simulink library "per"  (Simulink 8.2)
settings: Solver=ode45  StartTime=0.0  StopTime=10.0  RelTol=1e-3
undefined symbols (not defined in the file or in its folder): C_TICK_TIME_S, ENUM_LANEQUALITY_HIGH, ENUM_LANEQUALITY_MEDIUM, ENUM_SENSORSTATE_NORMAL, FALSE, KAPP_VehicleWidth_m, KPER_C0CrossingThr_m, KPER_CalDefaultTLC_s, KPER_CalTLCMax_s, KPER_CalTLCMin_s, KPER_DefaultLaneWidth_m, KPER_LaneWidHoldOnTime_s, KPER_LaneWidRampFinErrThres_m, KPER_LaneWidRampFinTimeThres_s, KPER_LaneWidRampInFalRt_mps, KPER_LaneWidRampInRisRt_mps, KPER_LaneWidRampOutFalRt_mps, KPER_LaneWidRampOutRisRt_mps, KPER_TLCDefaultValue_s, KPER_UseCalTLC_flg, TRUE
libraries: hcu_lib x16, cam x1, rad x1, sdf x1
(part 1 of 2)
settings Model: Creator=xsellart  LastModifiedBy=14069

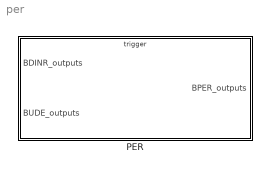
== system per ==
  PER : Subsystem

== system per/PER ==
  BDINR_outputs : Inport  OutDataTypeStr=Bus: BDINR_outputs
  BUDE_outputs : Inport  Port=2  OutDataTypeStr=Bus: BUDE_outputs
  trig_PER : TriggerPort  TriggerType=function-call
      settings: AttributesFormatString=State = %<StatesWhenEnabling>
  Bus Creator : BusCreator  Inputs=37  OutDataTypeStr=Bus: BPER_outputs
  Bus Selector1 : BusSelector  OutputSignals=VDINR_CamInternalError_flg,VDINR_LaneQualityL_enum,VDINR_LaneQualityR_enum,VDINR_LaneC0L_m,VDINR_LaneC0R_m,VDINR_LaneC1L_rad,VDINR_LaneC1R_rad,VDINR_LaneC2L_rat,VDINR_LaneC2R_rat,VDINR_LaneC3L_rat,VDINR_LaneC3R_rat,VDINR_TLCL_s,VDINR_TLCLValid_flg,VDINR_TLCR_s,VDINR_TLCRValid_flg,VDINR_VehSpd_mps,VDINR_YawRate_radps,VDINR_ViewRangeEndL_m,VDINR_ViewRangeEndR_m
  Bus Selector2 : BusSelector  OutputSignals=VUDE_NOFTRACKS_num,VUDE_TRACKSX_m,VUDE_TRACKSY_m,VUDE_TRACKSOBST_enum,VUDE_TRACKSVEL_mps,VUDE_TRACKSWIDTH_m,VUDE_TRACKSID_enum,VUDE_TRACKSATT_rad,VUDE_TRACKSEXSPROB_num,VUDE_TRACKSACCEL_mps2,VUDE_RadObjectValid_flg,VUDE_TRACKSRADDYNSTAT_enum,VUDE_CamObstacleValid_flg,VUDE_TRACKSMEDYNSTAT_enum
  per : Subsystem
  BPER_outputs : Outport  OutDataTypeStr=Bus: BPER_outputs
  wires:
  BDINR_outputs/1 -> Bus Selector1/1
  BUDE_outputs/1 -> Bus Selector2/1
  Bus Creator/1 -> BPER_outputs/1  "BPER_outputs"
  Bus Selector2/1 -> per/20(VUDE_NOfTracks_num)  "<VUDE_NOFTRACKS_num>"
  Bus Selector2/2 -> per/21(VUDE_TracksX_num)  "<VUDE_TRACKSX_m>"
  Bus Selector2/6 -> per/25(VUDE_TracksWidth_m)  "<VUDE_TRACKSWIDTH_m>"
  Bus Selector2/3 -> per/22(VUDE_TracksY_num)  "<VUDE_TRACKSY_m>"
  Bus Selector2/4 -> per/23(VUDE_TracksObsType_num)  "<VUDE_TRACKSOBST_enum>"
  Bus Selector2/5 -> per/24(VUDE_TracksVel_mps)  "<VUDE_TRACKSVEL_mps>"
  per/6(VPER_TargTypeVect30_enum) -> Bus Creator/6
  per/8(VPER_TargWidthVect30_m) -> Bus Creator/8
  per/7(VPER_TargAbsSpeedVect30_mps) -> Bus Creator/7
  per/5(VPER_TargYPosVect30_m) -> Bus Creator/5
  per/2(VPER_RadarStatus_enum) -> Bus Creator/2
  per/1(VPER_CameraStatus_enum) -> Bus Creator/1
  per/12(VPER_FusionStatus_enum) -> Bus Creator/12
  per/3(VPER_NumberOfTargets_enum) -> Bus Creator/3
  per/4(VPER_TargXPosVect30_m) -> Bus Creator/4
  Bus Selector2/7 -> per/26(VUDE_TracksId_num)  "<VUDE_TRACKSID_enum>"
  Bus Selector2/8 -> per/27(VUDE_TracksAtt_rad)  "<VUDE_TRACKSATT_rad>"
  Bus Selector2/9 -> per/28(VUDE_TracksExisProb_num)  "<VUDE_TRACKSEXSPROB_num>"
  per/9(VPER_TargIdVect30_num) -> Bus Creator/9
  per/10(VPER_TargAttitudeVect30_rad) -> Bus Creator/10
  per/11(VPER_TargExistProbVect30_num) -> Bus Creator/11
  Bus Selector2/10 -> per/29(VUDE_TracksAccel_mps2)  "<VUDE_TRACKSACCEL_mps2>"
  per/13(VPER_TargAccelVect30_mps2) -> Bus Creator/13
  Bus Selector2/11 -> per/30(VUDE_RadObjectValid_flg)  "<VUDE_RadObjectValid_flg>"
  Bus Selector2/12 -> per/31(VUDE_TRACKSRADDYNSTAT_enum)  "<VUDE_TRACKSRADDYNSTAT_enum>"
  Bus Selector2/13 -> per/32(VUDE_CamObstacleValid_flg)  "<VUDE_CamObstacleValid_flg>"
  Bus Selector2/14 -> per/33(VUDE_TRACKSMEDYNSTAT_enum)  "<VUDE_TRACKSMEDYNSTAT_enum>"
  per/14(VPER_RadObjValidVect30_flg) -> Bus Creator/14
  per/15(VPER_RadDynPropertyVect30_enum) -> Bus Creator/15
  per/16(VPER_CamObsValidVect30_flg) -> Bus Creator/16
  per/17(VPER_CamObsStatusVect30_enum) -> Bus Creator/17
  Bus Selector1/11 -> per/11(VDINR_LaneC3R_rat)  "<VDINR_LaneC3R_rat>"
  Bus Selector1/15 -> per/15(VDINR_TLCRValid_fig)  "<VDINR_TLCRValid_flg>"
  Bus Selector1/12 -> per/12(VDINR_TLCL_s)  "<VDINR_TLCL_s>"
  Bus Selector1/14 -> per/14(VDINR_TLCR_s)  "<VDINR_TLCR_s>"
  Bus Selector1/13 -> per/13(VDINR_TLCLValid_fig)  "<VDINR_TLCLValid_flg>"
  Bus Selector1/16 -> per/16(VDINR_VehSpd_mps)  "<VDINR_VehSpd_mps>"
  Bus Selector1/18 -> per/18(VDINR_ViewRangeEndL_m)  "<VDINR_ViewRangeEndL_m>"
  Bus Selector1/17 -> per/17(VDINR_YawRate_radps)  "<VDINR_YawRate_radps>"
  Bus Selector1/19 -> per/19(VDINR_ViewRangeEndR_m)  "<VDINR_ViewRangeEndR_m>"
  per/18(VPER_LeftLaneAvail_fig) -> Bus Creator/18
  per/19(VPER_RightLaneAvail_fig) -> Bus Creator/19
  per/20(VPER_CenterLineC0_m) -> Bus Creator/20
  per/21(VPER_CenterLineC1_rad) -> Bus Creator/21
  per/22(VPER_CenterLineC2_rat) -> Bus Creator/22
  per/23(VPER_CenterLineC3_rat) -> Bus Creator/23
  per/24(VPER_LaneC0L_m) -> Bus Creator/24
  per/25(VPER_LaneC1L_rad) -> Bus Creator/25
  per/26(VPER_LaneC2L_rat) -> Bus Creator/26
  per/27(VPER_LaneC3L_rat) -> Bus Creator/27
  per/28(VPER_LaneC0R_m) -> Bus Creator/28
  per/29(VPER_LaneC1R_rad) -> Bus Creator/29
  per/30(VPER_LaneC2R_rat) -> Bus Creator/30
  per/31(VPER_LaneC3R_rat) -> Bus Creator/31
  per/32(VPER_TLCL_s) -> Bus Creator/32
  per/33(VPER_TLCR_s) -> Bus Creator/33
  per/34(VPER_C1LBias_rad) -> Bus Creator/34
  per/35(VPER_C1RBias_rad) -> Bus Creator/35
  per/36(VPER_ResidualLaneL_s) -> Bus Creator/36
  per/37(VPER_ResidualLaneR_s) -> Bus Creator/37
  Bus Selector1/1 -> per/1(VDINR_CamInternalError_flg)  "<VDINR_CamInternalError_flg>"
  Bus Selector1/2 -> per/2(VDINR_LaneQualityL_enum)  "<VDINR_LaneQualityL_enum>"
  Bus Selector1/3 -> per/3(VDINR_LaneQualityR_enum)  "<VDINR_LaneQualityR_enum>"
  Bus Selector1/4 -> per/4(VDINR_LaneC0L_m)  "<VDINR_LaneC0L_m>"
  Bus Selector1/5 -> per/5(VDINR_LaneC0R_m)  "<VDINR_LaneC0R_m>"
  Bus Selector1/6 -> per/6(VDINR_LaneC1L_rad)  "<VDINR_LaneC1L_rad>"
  Bus Selector1/7 -> per/7(VDINR_LaneC1R_rad)  "<VDINR_LaneC1R_rad>"
  Bus Selector1/8 -> per/8(VDINR_LaneC2L_rat)  "<VDINR_LaneC2L_rat>"
  Bus Selector1/9 -> per/9(VDINR_LaneC2R_rat)  "<VDINR_LaneC2R_rat>"
  Bus Selector1/10 -> per/10(VDINR_LaneC3L_rat)  "<VDINR_LaneC3L_rat>"

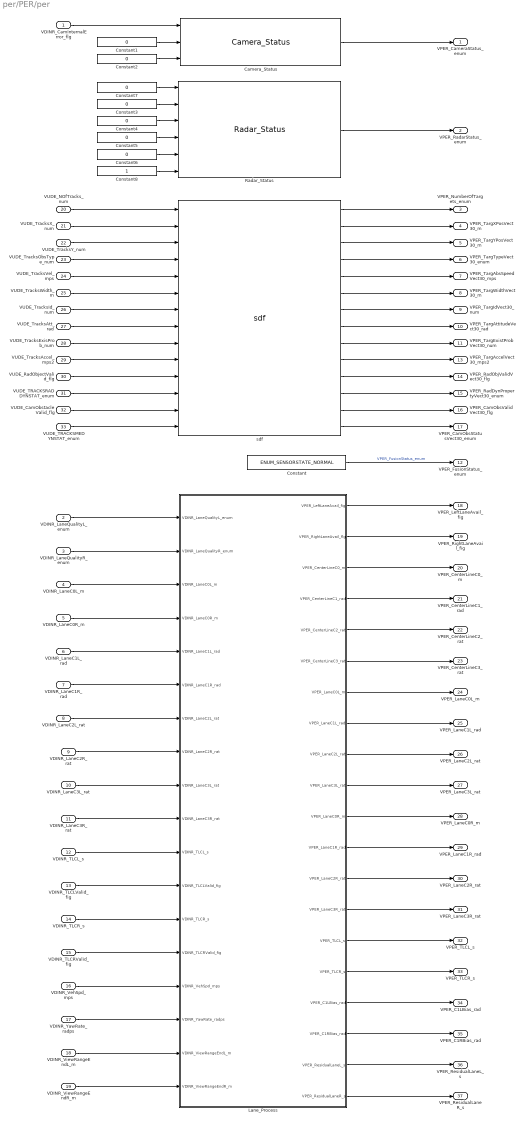
== system per/PER/per ==
  VDINR_CamInternalError_flg : Inport
  VDINR_LaneQualityL_enum : Inport  Port=2
  VDINR_LaneQualityR_enum : Inport  Port=3
  VDINR_LaneC0L_m : Inport  Port=4
  VDINR_LaneC0R_m : Inport  Port=5
  VDINR_LaneC1L_rad : Inport  Port=6
  VDINR_LaneC1R_rad : Inport  Port=7
  VDINR_LaneC2L_rat : Inport  Port=8
  VDINR_LaneC2R_rat : Inport  Port=9
  VDINR_LaneC3L_rat : Inport  Port=10
  VDINR_LaneC3R_rat : Inport  Port=11
  VDINR_TLCL_s : Inport  Port=12
  VDINR_TLCLValid_fig : Inport  Port=13
  VDINR_TLCR_s : Inport  Port=14
  VDINR_TLCRValid_fig : Inport  Port=15
  VDINR_VehSpd_mps : Inport  Port=16
  VDINR_YawRate_radps : Inport  Port=17
  VDINR_ViewRangeEndL_m : Inport  Port=18
  VDINR_ViewRangeEndR_m : Inport  Port=19
  VUDE_NOfTracks_num : Inport  Port=20
  VUDE_TracksX_num : Inport  Port=21
  VUDE_TracksY_num : Inport  Port=22
  VUDE_TracksObsType_num : Inport  Port=23
  VUDE_TracksVel_mps : Inport  Port=24
  VUDE_TracksWidth_m : Inport  Port=25
  VUDE_TracksId_num : Inport  Port=26
  VUDE_TracksAtt_rad : Inport  Port=27
  VUDE_TracksExisProb_num : Inport  Port=28
  VUDE_TracksAccel_mps2 : Inport  Port=29
  VUDE_RadObjectValid_flg : Inport  Port=30
  VUDE_TRACKSRADDYNSTAT_enum : Inport  Port=31
  VUDE_CamObstacleValid_flg : Inport  Port=32
  VUDE_TRACKSMEDYNSTAT_enum : Inport  Port=33
  Camera_Status : cam/Camera_Status
  Constant : Constant  Value=ENUM_SENSORSTATE_NORMAL  OutDataTypeStr=uint8
  Constant{1..7} (7 alike) : Constant  Value=0  OutDataTypeStr=boolean
  Constant8 : Constant  OutDataTypeStr=boolean
  Lane_Process : Subsystem  TreatAsAtomicUnit=on
  Radar_Status : rad/Radar_Status
  sdf : sdf/sdf
  VPER_CameraStatus_enum : Outport
  VPER_RadarStatus_enum : Outport  Port=2
  VPER_NumberOfTargets_enum : Outport  Port=3
  VPER_TargXPosVect30_m : Outport  Port=4
  VPER_TargYPosVect30_m : Outport  Port=5
  VPER_TargTypeVect30_enum : Outport  Port=6
  VPER_TargAbsSpeedVect30_mps : Outport  Port=7
  VPER_TargWidthVect30_m : Outport  Port=8
  VPER_TargIdVect30_num : Outport  Port=9
  VPER_TargAttitudeVect30_rad : Outport  Port=10
  VPER_TargExistProbVect30_num : Outport  Port=11
  VPER_FusionStatus_enum : Outport  Port=12
  VPER_TargAccelVect30_mps2 : Outport  Port=13
  VPER_RadObjValidVect30_flg : Outport  Port=14
  VPER_RadDynPropertyVect30_enum : Outport  Port=15
  VPER_CamObsValidVect30_flg : Outport  Port=16
  VPER_CamObsStatusVect30_enum : Outport  Port=17
  VPER_LeftLaneAvail_fig : Outport  Port=18
  VPER_RightLaneAvail_fig : Outport  Port=19
  VPER_CenterLineC0_m : Outport  Port=20
  VPER_CenterLineC1_rad : Outport  Port=21
  VPER_CenterLineC2_rat : Outport  Port=22
  VPER_CenterLineC3_rat : Outport  Port=23
  VPER_LaneC0L_m : Outport  Port=24
  VPER_LaneC1L_rad : Outport  Port=25
  VPER_LaneC2L_rat : Outport  Port=26
  VPER_LaneC3L_rat : Outport  Port=27
  VPER_LaneC0R_m : Outport  Port=28
  VPER_LaneC1R_rad : Outport  Port=29
  VPER_LaneC2R_rat : Outport  Port=30
  VPER_LaneC3R_rat : Outport  Port=31
  VPER_TLCL_s : Outport  Port=32
  VPER_TLCR_s : Outport  Port=33
  VPER_C1LBias_rad : Outport  Port=34
  VPER_C1RBias_rad : Outport  Port=35
  VPER_ResidualLaneL_s : Outport  Port=36
  VPER_ResidualLaneR_s : Outport  Port=37
  wires:
  Constant/1 -> VPER_FusionStatus_enum/1  "VPER_FusionStatus_enum"
  sdf/6 -> VPER_TargWidthVect30_m/1
  sdf/5 -> VPER_TargAbsSpeedVect30_mps/1
  sdf/4 -> VPER_TargTypeVect30_enum/1
  sdf/3 -> VPER_TargYPosVect30_m/1
  sdf/2 -> VPER_TargXPosVect30_m/1
  sdf/1 -> VPER_NumberOfTargets_enum/1
  Radar_Status/1 -> VPER_RadarStatus_enum/1
  VUDE_TracksWidth_m/1 -> sdf/6
  VUDE_NOfTracks_num/1 -> sdf/1
  Camera_Status/1 -> VPER_CameraStatus_enum/1
  VUDE_TracksVel_mps/1 -> sdf/5
  VDINR_CamInternalError_flg/1 -> Camera_Status/1
  VUDE_TracksObsType_num/1 -> sdf/4
  VUDE_TracksX_num/1 -> sdf/2
  Constant1/1 -> Camera_Status/2
  Constant2/1 -> Camera_Status/3
  VUDE_TracksY_num/1 -> sdf/3
  VUDE_TracksId_num/1 -> sdf/7
  VUDE_TracksAtt_rad/1 -> sdf/8
  VUDE_TracksExisProb_num/1 -> sdf/9
  sdf/7 -> VPER_TargIdVect30_num/1
  sdf/8 -> VPER_TargAttitudeVect30_rad/1
  sdf/9 -> VPER_TargExistProbVect30_num/1
  sdf/10 -> VPER_TargAccelVect30_mps2/1
  VUDE_TracksAccel_mps2/1 -> sdf/10
  VUDE_RadObjectValid_flg/1 -> sdf/11
  VUDE_TRACKSRADDYNSTAT_enum/1 -> sdf/12
  VUDE_CamObstacleValid_flg/1 -> sdf/13
  VUDE_TRACKSMEDYNSTAT_enum/1 -> sdf/14
  sdf/11 -> VPER_RadObjValidVect30_flg/1
  sdf/12 -> VPER_RadDynPropertyVect30_enum/1
  sdf/13 -> VPER_CamObsValidVect30_flg/1
  sdf/14 -> VPER_CamObsStatusVect30_enum/1
  VDINR_LaneQualityR_enum/1 -> Lane_Process/2(VDINR_LaneQualityR_enum)
  VDINR_LaneQualityL_enum/1 -> Lane_Process/1(VDINR_LaneQualityL_enum)
  VDINR_LaneC0L_m/1 -> Lane_Process/3(VDINR_LaneC0L_m)
  VDINR_LaneC0R_m/1 -> Lane_Process/4(VDINR_LaneC0R_m)
  VDINR_LaneC1L_rad/1 -> Lane_Process/5(VDINR_LaneC1L_rad)
  VDINR_LaneC1R_rad/1 -> Lane_Process/6(VDINR_LaneC1R_rad)
  VDINR_LaneC2L_rat/1 -> Lane_Process/7(VDINR_LaneC2L_rat)
  VDINR_LaneC2R_rat/1 -> Lane_Process/8(VDINR_LaneC2R_rat)
  VDINR_LaneC3L_rat/1 -> Lane_Process/9(VDINR_LaneC3L_rat)
  VDINR_LaneC3R_rat/1 -> Lane_Process/10(VDINR_LaneC3R_rat)
  VDINR_TLCL_s/1 -> Lane_Process/11(VDINR_TLCL_s)
  VDINR_TLCLValid_fig/1 -> Lane_Process/12(VDINR_TLCLValid_fig)
  VDINR_TLCR_s/1 -> Lane_Process/13(VDINR_TLCR_s)
  VDINR_TLCRValid_fig/1 -> Lane_Process/14(VDINR_TLCRValid_fig)
  VDINR_VehSpd_mps/1 -> Lane_Process/15(VDINR_VehSpd_mps)
  Lane_Process/16(VPER_TLCR_s) -> VPER_TLCR_s/1
  Lane_Process/15(VPER_TLCL_s) -> VPER_TLCL_s/1
  Lane_Process/14(VPER_LaneC3R_rat) -> VPER_LaneC3R_rat/1
  Lane_Process/13(VPER_LaneC2R_rat) -> VPER_LaneC2R_rat/1
  Lane_Process/12(VPER_LaneC1R_rad) -> VPER_LaneC1R_rad/1
  Lane_Process/11(VPER_LaneC0R_m) -> VPER_LaneC0R_m/1
  Lane_Process/10(VPER_LaneC3L_rat) -> VPER_LaneC3L_rat/1
  Lane_Process/9(VPER_LaneC2L_rat) -> VPER_LaneC2L_rat/1
  Lane_Process/8(VPER_LaneC1L_rad) -> VPER_LaneC1L_rad/1
  Lane_Process/7(VPER_LaneC0L_m) -> VPER_LaneC0L_m/1
  Lane_Process/6(VPER_CenterLineC3_rat) -> VPER_CenterLineC3_rat/1
  Lane_Process/5(VPER_CenterLineC2_rat) -> VPER_CenterLineC2_rat/1
  Lane_Process/4(VPER_CenterLineC1_rad) -> VPER_CenterLineC1_rad/1
  Lane_Process/3("VPER_CenterLineC0_m ") -> VPER_CenterLineC0_m/1
  Lane_Process/1(VPER_LeftLaneAvail_fig) -> VPER_LeftLaneAvail_fig/1
  Lane_Process/2(VPER_RightLaneAvail_flg) -> VPER_RightLaneAvail_fig/1
  VDINR_YawRate_radps/1 -> Lane_Process/16(VDINR_YawRate_radps)
  VDINR_ViewRangeEndL_m/1 -> Lane_Process/17(VDINR_ViewRangeEndL_m)
  VDINR_ViewRangeEndR_m/1 -> Lane_Process/18(VDINR_ViewRangeEndR_m)
  Lane_Process/17(VPER_C1LBias_rad) -> VPER_C1LBias_rad/1
  Lane_Process/18(VPER_C1RBias_rad) -> VPER_C1RBias_rad/1
  Lane_Process/19(VPER_ResidualLaneL_s) -> VPER_ResidualLaneL_s/1
  Lane_Process/20(VPER_ResidualLaneR_s) -> VPER_ResidualLaneR_s/1
  Constant3/1 -> Radar_Status/2
  Constant4/1 -> Radar_Status/3
  Constant5/1 -> Radar_Status/4
  Constant6/1 -> Radar_Status/5
  Constant7/1 -> Radar_Status/1
  Constant8/1 -> Radar_Status/6

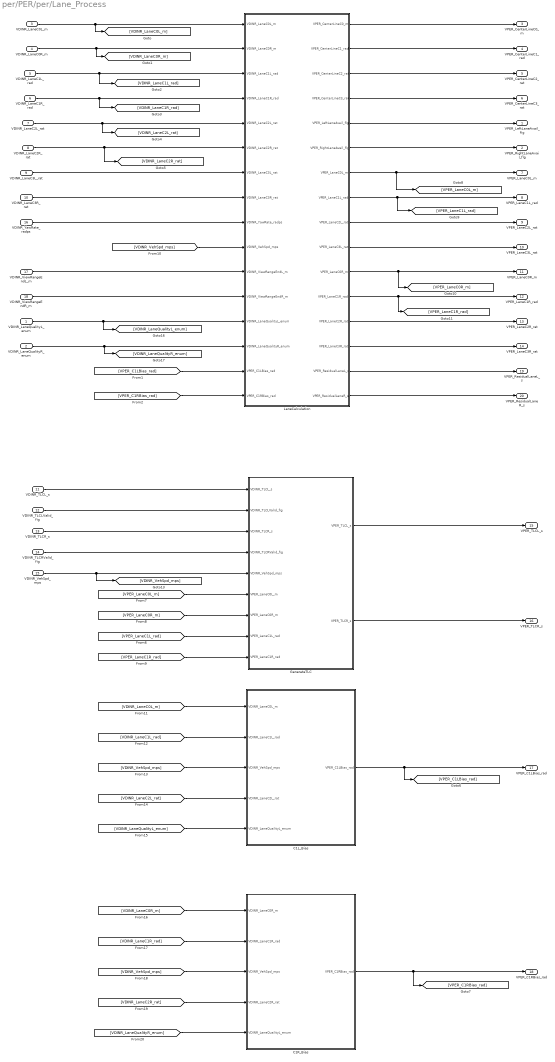
== system per/PER/per/Lane_Process ==
  VDINR_LaneQualityL_enum : Inport
  VDINR_LaneQualityR_enum : Inport  Port=2
  VDINR_LaneC0L_m : Inport  Port=3
  VDINR_LaneC0R_m : Inport  Port=4
  VDINR_LaneC1L_rad : Inport  Port=5
  VDINR_LaneC1R_rad : Inport  Port=6
  VDINR_LaneC2L_rat : Inport  Port=7
  VDINR_LaneC2R_rat : Inport  Port=8
  VDINR_LaneC3L_rat : Inport  Port=9
  VDINR_LaneC3R_rat : Inport  Port=10
  VDINR_TLCL_s : Inport  Port=11
  VDINR_TLCLValid_fig : Inport  Port=12
  VDINR_TLCR_s : Inport  Port=13
  VDINR_TLCRValid_fig : Inport  Port=14
  VDINR_VehSpd_mps : Inport  Port=15
  VDINR_YawRate_radps : Inport  Port=16
  VDINR_ViewRangeEndL_m : Inport  Port=17
  VDINR_ViewRangeEndR_m : Inport  Port=18
  C1L_Bias : Subsystem  TreatAsAtomicUnit=on
  C1R_Bias : Subsystem  TreatAsAtomicUnit=on
  GenerateTLC : Subsystem
  LaneCalculation : Subsystem
  VPER_LeftLaneAvail_fig : Outport
  VPER_RightLaneAvail_flg : Outport  Port=2
  "VPER_CenterLineC0_m " : Outport  Port=3
  VPER_CenterLineC1_rad : Outport  Port=4
  VPER_CenterLineC2_rat : Outport  Port=5
  VPER_CenterLineC3_rat : Outport  Port=6
  VPER_LaneC0L_m : Outport  Port=7
  VPER_LaneC1L_rad : Outport  Port=8
  VPER_LaneC2L_rat : Outport  Port=9
  VPER_LaneC3L_rat : Outport  Port=10
  VPER_LaneC0R_m : Outport  Port=11
  VPER_LaneC1R_rad : Outport  Port=12
  VPER_LaneC2R_rat : Outport  Port=13
  VPER_LaneC3R_rat : Outport  Port=14
  VPER_TLCL_s : Outport  Port=15
  VPER_TLCR_s : Outport  Port=16
  VPER_C1LBias_rad : Outport  Port=17
  VPER_C1RBias_rad : Outport  Port=18
  VPER_ResidualLaneL_s : Outport  Port=19
  VPER_ResidualLaneR_s : Outport  Port=20
  wires:
  VDINR_LaneC1L_rad/1 -> [VDINR_LaneC1L_rad], LaneCalculation/3(VDINR_LaneC1L_rad)
  VDINR_LaneC2L_rat/1 -> [VDINR_LaneC2L_rat], LaneCalculation/5(VDINR_LaneC2L_rat)
  VDINR_LaneC2R_rat/1 -> [VDINR_LaneC2R_rat], LaneCalculation/6(VDINR_LaneC2R_rat)
  VDINR_LaneC3L_rat/1 -> LaneCalculation/7(VDINR_LaneC3L_rat)
  VDINR_LaneC3R_rat/1 -> LaneCalculation/8(VDINR_LaneC3R_rat)
  VDINR_LaneQualityL_enum/1 -> [VDINR_LaneQualityL_enum], LaneCalculation/13(VDINR_LaneQualityL_enum)
  LaneCalculation/1("VPER_CenterLineC0_m ") -> "VPER_CenterLineC0_m "/1
  LaneCalculation/2(VPER_CenterLineC1_rad) -> VPER_CenterLineC1_rad/1
  LaneCalculation/3(VPER_CenterLineC2_rat) -> VPER_CenterLineC2_rat/1
  LaneCalculation/4(VPER_CenterLineC3_rat) -> VPER_CenterLineC3_rat/1
  VDINR_TLCL_s/1 -> GenerateTLC/1(VDINR_TLCL_s)
  VDINR_TLCLValid_fig/1 -> GenerateTLC/2(VDINR_TLCLValid_fig)
  VDINR_TLCR_s/1 -> GenerateTLC/3(VDINR_TLCR_s)
  VDINR_TLCRValid_fig/1 -> GenerateTLC/4(VDINR_TLCRValid_fig)
  GenerateTLC/1(VPER_TLCL_s) -> VPER_TLCL_s/1
  GenerateTLC/2(VPER_TLCR_s) -> VPER_TLCR_s/1
  [VPER_LaneC1L_rad] -> GenerateTLC/8(VPER_LaneC1L_rad)
  [VPER_LaneC0L_m] -> GenerateTLC/6(VPER_LaneC0L_m)
  [VPER_LaneC0R_m] -> GenerateTLC/7(VPER_LaneC0R_m)
  VDINR_VehSpd_mps/1 -> [VDINR_VehSpd_mps], GenerateTLC/5(VDINR_VehSpd_mps)
  [VPER_LaneC1R_rad] -> GenerateTLC/9(VPER_LaneC1R_rad)
  VDINR_YawRate_radps/1 -> LaneCalculation/9(VDINR_YawRate_radps)
  [VDINR_VehSpd_mps] -> LaneCalculation/10(VDINR_VehSpd_mps)
  VDINR_ViewRangeEndL_m/1 -> LaneCalculation/11(VDINR_ViewRangeEndL_m)
  VDINR_ViewRangeEndR_m/1 -> LaneCalculation/12(VDINR_ViewRangeEndR_m)
  LaneCalculation/5(VPER_LeftLaneAvail_flg) -> VPER_LeftLaneAvail_fig/1
  LaneCalculation/6(VPER_RightLaneAvail_flg) -> VPER_RightLaneAvail_flg/1
  [VDINR_LaneC0L_m] -> C1L_Bias/1(VDINR_LaneC0L_m)
  [VDINR_VehSpd_mps] -> C1L_Bias/3(VDINR_VehSpd_mps)
  [VDINR_LaneC2L_rat] -> C1L_Bias/4(VDINR_LaneC2L_rat)
  [VDINR_LaneQualityL_enum] -> C1L_Bias/5(VDINR_LaneQualityL_enum)
  C1L_Bias/1(VPER_C1LBias_rad) -> [VPER_C1LBias_rad], VPER_C1LBias_rad/1
  C1R_Bias/1(VPER_C1RBias_rad) -> [VPER_C1RBias_rad], VPER_C1RBias_rad/1
  [VDINR_LaneQualityR_enum] -> C1R_Bias/5(VDINR_LaneQualityL_enum)
  [VDINR_LaneC0R_m] -> C1R_Bias/1(VDINR_LaneC0R_m)
  [VDINR_VehSpd_mps] -> C1R_Bias/3(VDINR_VehSpd_mps)
  [VDINR_LaneC2R_rat] -> C1R_Bias/4(VDINR_LaneC2R_rat)
  VDINR_LaneC1R_rad/1 -> [VDINR_LaneC1R_rad], LaneCalculation/4(VDINR_LaneC1R_rad)
  LaneCalculation/7(VPER_LaneC0L_m) -> [VPER_LaneC0L_m], VPER_LaneC0L_m/1
  LaneCalculation/8(VPER_LaneC1L_rad) -> [VPER_LaneC1L_rad], VPER_LaneC1L_rad/1
  LaneCalculation/9(VPER_LaneC2L_rat) -> VPER_LaneC2L_rat/1
  LaneCalculation/10(VPER_LaneC3L_rat) -> VPER_LaneC3L_rat/1
  LaneCalculation/11(VPER_LaneC0R_m) -> [VPER_LaneC0R_m], VPER_LaneC0R_m/1
  LaneCalculation/12(VPER_LaneC1R_rad) -> [VPER_LaneC1R_rad], VPER_LaneC1R_rad/1
  LaneCalculation/13(VPER_LaneC2R_rat) -> VPER_LaneC2R_rat/1
  LaneCalculation/14(VPER_LaneC3R_rat) -> VPER_LaneC3R_rat/1
  VDINR_LaneQualityR_enum/1 -> [VDINR_LaneQualityR_enum], LaneCalculation/14(VDINR_LaneQualityR_enum)
  VDINR_LaneC0L_m/1 -> LaneCalculation/1(VDINR_LaneC0L_m), [VDINR_LaneC0L_m]
  VDINR_LaneC0R_m/1 -> [VDINR_LaneC0R_m], LaneCalculation/2(VDINR_LaneC0R_m)
  [VDINR_LaneC1R_rad] -> C1R_Bias/2(VDINR_LaneC1R_rad)
  [VDINR_LaneC1L_rad] -> C1L_Bias/2(VDINR_LaneC1L_rad)
  [VPER_C1LBias_rad] -> LaneCalculation/15(VPER_C1LBias_rad)
  [VPER_C1RBias_rad] -> LaneCalculation/16(VPER_C1RBias_rad)
  LaneCalculation/15(VPER_ResidualLaneL_s) -> VPER_ResidualLaneL_s/1
  LaneCalculation/16(VPER_ResidualLaneR_s) -> VPER_ResidualLaneR_s/1

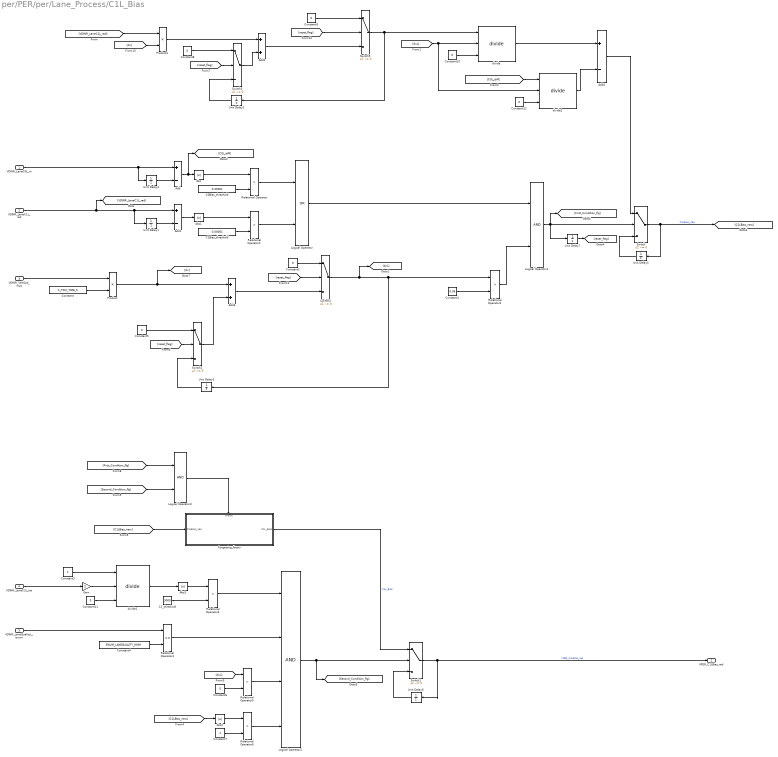
== system per/PER/per/Lane_Process/C1L_Bias ==
  VDINR_LaneC0L_m : Inport
  VDINR_LaneC1L_rad : Inport  Port=2
  VDINR_VehSpd_mps : Inport  Port=3
  VDINR_LaneC2L_rat : Inport  Port=4
  VDINR_LaneQualityL_enum : Inport  Port=5
  Abs{,1..3} (4 alike) : Abs
  Add : Sum  Inputs=+-
  Add1 : Sum  Inputs=+-
  Add2 : Sum
  Add3 : Sum
  Add4 : Sum  Inputs=+-
  C0Bias_threshold : Constant  Value=0.00001  OutDataTypeStr=single
  C1Bias_threshold : Constant  Value=0.00001  OutDataTypeStr=single
  C2_threshold : Constant  Value=3000  OutDataTypeStr=single
  Constant : Constant  Value=C_TICK_TIME_S
  Constant1 : Constant  Value=0.04  OutDataTypeStr=single
  Constant{2,5,8..12} (7 alike) : Constant  Value=0  OutDataTypeStr=single
  Constant3 : Constant  OutDataTypeStr=single
  Constant4 : Constant  Value=ENUM_LANEQUALITY_HIGH
  Constant6 : Constant  Value=5  OutDataTypeStr=single
  Constant7 : Constant  OutDataTypeStr=single
  Forgetting_factor : Subsystem  TreatAsAtomicUnit=on
  Gain : Gain  Gain=2
  Logical Operator : Logic  Operator=OR  AllPortsSameDT=off  OutDataTypeStr=boolean
  Logical Operator1 : Logic  AllPortsSameDT=off  OutDataTypeStr=boolean
  Logical Operator2 : Logic  Inputs=4  AllPortsSameDT=off  OutDataTypeStr=boolean
  Logical Operator3 : Logic  AllPortsSameDT=off  OutDataTypeStr=boolean
  Product : Product
  Product1 : Product
  Relational Operator{,1..3} (4 alike) : RelationalOperator  Operator=>  OutDataTypeStr=boolean
  Relational Operator4 : RelationalOperator  Operator===  OutDataTypeStr=boolean
  Relational Operator5 : RelationalOperator  Operator=<  OutDataTypeStr=boolean
  Relational Operator6 : RelationalOperator  Operator=<  OutDataTypeStr=boolean
  Switch{,1..5} (6 alike) : Switch  Criteria=u2 ~= 0
  Unit Delay{1..7} (7 alike) : UnitDelay  SampleTime=-1
  divide : hcu_lib/divide
  divide1 : hcu_lib/divide
  divide2 : hcu_lib/divide
  VPER_C1LBias_rad : Outport
  wires:
  VDINR_LaneC0L_m/1 -> Unit Delay4/1, Add/1
  Unit Delay4/1 -> Add/2
  VDINR_LaneC1L_rad/1 -> [VDINR_LaneC1L_rad], Unit Delay1/1, Add1/1
  Unit Delay1/1 -> Add1/2
  Add/1 -> [C0L_diff], Abs/1
  Add1/1 -> Abs1/1
  VDINR_VehSpd_mps/1 -> Product/1
  Abs/1 -> Relational Operator/1
  C0Bias_threshold/1 -> Relational Operator/2
  Abs1/1 -> Relational Operator1/1
  C1Bias_threshold/1 -> Relational Operator1/2
  Add3/1 -> Switch4/3
  Constant1/1 -> Relational Operator2/2
  Relational Operator/1 -> Logical Operator/1
  Relational Operator1/1 -> Logical Operator/2
  Logical Operator/1 -> Logical Operator1/1
  Relational Operator2/1 -> Logical Operator1/2
  Logical Operator1/1 -> Switch/2, [First_Condition_flg], Unit Delay7/1
  [dx] -> Product1/2
  [VDINR_LaneC1L_rad] -> Product1/1
  Product1/1 -> Add2/1
  Constant/1 -> Product/2
  Product/1 -> [dx], Add3/1
  [dxL] -> divide2/2, divide/2
  divide/1 -> Add4/1
  [C0L_diff] -> divide2/1
  divide2/1 -> Add4/2
  Add4/1 -> Switch/1
  VDINR_LaneC2L_rat/1 -> Gain/1
  C2_threshold/1 -> Relational Operator3/2
  VDINR_LaneQualityL_enum/1 -> Relational Operator4/1
  Constant4/1 -> Relational Operator4/2
  Relational Operator3/1 -> Logical Operator2/1
  Relational Operator4/1 -> Logical Operator2/2
  [dxL] -> Relational Operator5/1
  Constant6/1 -> Relational Operator5/2
  Relational Operator5/1 -> Logical Operator2/3
  Relational Operator6/1 -> Logical Operator2/4
  Switch/1 -> Unit Delay5/1, [C1LBias_new]  "C1LBias_new"
  Switch1/1 -> Unit Delay6/1, VPER_C1LBias_rad/1  "VPER_C1LBias_rad"
  [C1LBias_new] -> Abs2/1
  Abs2/1 -> Relational Operator6/1
  Constant7/1 -> Relational Operator6/2
  Forgetting_factor/1(C1L_Bias) -> Switch1/1  "C1L_Bias"
  [C1LBias_new] -> Forgetting_factor/1(C1LBias_new)
  Unit Delay5/1 -> Switch/3
  Unit Delay6/1 -> Switch1/3
  Abs3/1 -> Relational Operator3/1
  Logical Operator2/1 -> [Second_Condition_flg], Switch1/2
  Switch2/1 -> Add3/2
  Constant5/1 -> Switch2/1
  [reset_flag] -> Switch2/2
  Constant8/1 -> Switch3/1
  [reset_flag] -> Switch3/2
  Switch3/1 -> Add2/2
  Unit Delay7/1 -> [reset_flag]
  Unit Delay2/1 -> Switch3/3
  Unit Delay3/1 -> Switch2/3
  [First_Condition_flg] -> Logical Operator3/1
  [Second_Condition_flg] -> Logical Operator3/2
  Logical Operator3/1 -> Forgetting_factor/Enable
  [reset_flag] -> Switch4/2
  Constant2/1 -> Switch4/1
  Switch4/1 -> [dxL], Unit Delay3/1, Relational Operator2/1
  Add2/1 -> Switch5/3
  [reset_flag] -> Switch5/2
  Constant9/1 -> Switch5/1
  Switch5/1 -> divide/1, Unit Delay2/1
  Constant10/1 -> divide/3
  divide1/1 -> Abs3/1
  Constant3/1 -> divide1/1
  Gain/1 -> divide1/2
  Constant11/1 -> divide1/3
  Constant12/1 -> divide2/3

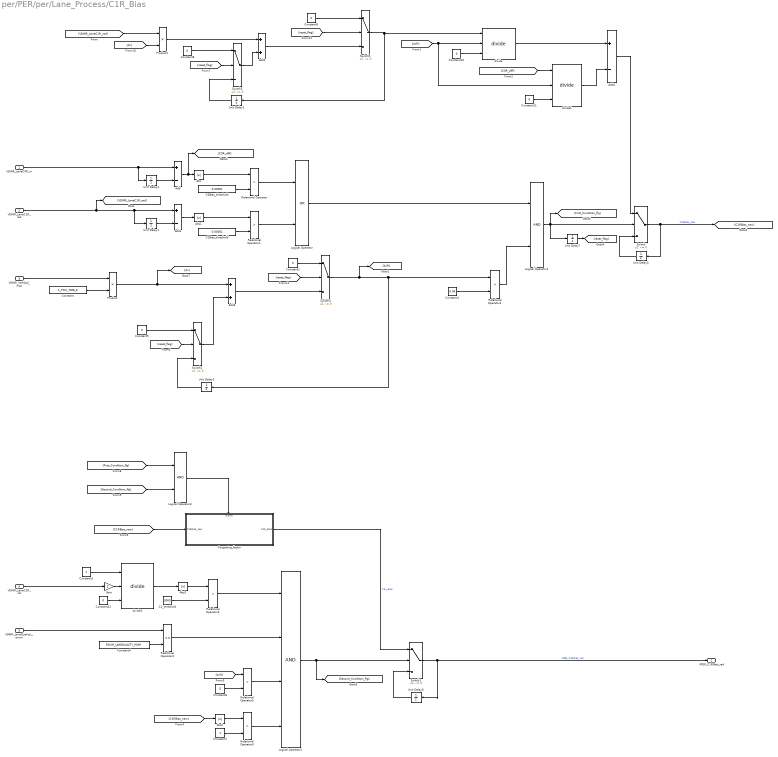
== system per/PER/per/Lane_Process/C1R_Bias ==
  VDINR_LaneC0R_m : Inport
  VDINR_LaneC1R_rad : Inport  Port=2
  VDINR_VehSpd_mps : Inport  Port=3
  VDINR_LaneC2R_rat : Inport  Port=4
  VDINR_LaneQualityL_enum : Inport  Port=5
  Abs{,1..3} (4 alike) : Abs
  Add : Sum  Inputs=+-
  Add1 : Sum  Inputs=+-
  Add2 : Sum
  Add3 : Sum
  Add4 : Sum  Inputs=+-
  C0Bias_threshold : Constant  Value=0.00001  OutDataTypeStr=single
  C1Bias_threshold : Constant  Value=0.00001  OutDataTypeStr=single
  C2_threshold : Constant  Value=3000  OutDataTypeStr=single
  Constant : Constant  Value=C_TICK_TIME_S
  Constant1 : Constant  Value=0.04  OutDataTypeStr=single
  Constant{2,5,8..12} (7 alike) : Constant  Value=0  OutDataTypeStr=single
  Constant3 : Constant  OutDataTypeStr=single
  Constant4 : Constant  Value=ENUM_LANEQUALITY_HIGH
  Constant6 : Constant  Value=5  OutDataTypeStr=single
  Constant7 : Constant  OutDataTypeStr=single
  Forgetting_factor : Subsystem  TreatAsAtomicUnit=on
  Gain : Gain  Gain=2
  Logical Operator : Logic  Operator=OR  AllPortsSameDT=off  OutDataTypeStr=boolean
  Logical Operator1 : Logic  AllPortsSameDT=off  OutDataTypeStr=boolean
  Logical Operator2 : Logic  Inputs=4  AllPortsSameDT=off  OutDataTypeStr=boolean
  Logical Operator3 : Logic  AllPortsSameDT=off  OutDataTypeStr=boolean
  Product : Product
  Product1 : Product
  Relational Operator{,1..3} (4 alike) : RelationalOperator  Operator=>  OutDataTypeStr=boolean
  Relational Operator4 : RelationalOperator  Operator===  OutDataTypeStr=boolean
  Relational Operator5 : RelationalOperator  Operator=<  OutDataTypeStr=boolean
  Relational Operator6 : RelationalOperator  Operator=<  OutDataTypeStr=boolean
  Switch{,1..5} (6 alike) : Switch  Criteria=u2 ~= 0
  Unit Delay{1..7} (7 alike) : UnitDelay  SampleTime=-1
  divide : hcu_lib/divide
  divide1 : hcu_lib/divide
  divide2 : hcu_lib/divide
  VPER_C1RBias_rad : Outport
  wires:
  VDINR_LaneC0R_m/1 -> Unit Delay4/1, Add/1
  Unit Delay4/1 -> Add/2
  VDINR_LaneC1R_rad/1 -> [VDINR_LaneC1R_rad], Unit Delay1/1, Add1/1
  Unit Delay1/1 -> Add1/2
  Add/1 -> [C0R_diff], Abs/1
  Add1/1 -> Abs1/1
  VDINR_VehSpd_mps/1 -> Product/1
  Abs/1 -> Relational Operator/1
  C0Bias_threshold/1 -> Relational Operator/2
  Abs1/1 -> Relational Operator1/1
  C1Bias_threshold/1 -> Relational Operator1/2
  Add3/1 -> Switch4/3
  Constant1/1 -> Relational Operator2/2
  Relational Operator/1 -> Logical Operator/1
  Relational Operator1/1 -> Logical Operator/2
  Logical Operator/1 -> Logical Operator1/1
  Relational Operator2/1 -> Logical Operator1/2
  Logical Operator1/1 -> Switch/2, [First_Condition_flg], Unit Delay7/1
  [dx] -> Product1/2
  [VDINR_LaneC1R_rad] -> Product1/1
  Product1/1 -> Add2/1
  Constant/1 -> Product/2
  Product/1 -> [dx], Add3/1
  [dxR] -> divide1/2, divide/2
  divide/1 -> Add4/1
  [C0R_diff] -> divide1/1
  divide1/1 -> Add4/2
  Add4/1 -> Switch/1
  VDINR_LaneC2R_rat/1 -> Gain/1
  divide2/1 -> Abs3/1
  C2_threshold/1 -> Relational Operator3/2
  VDINR_LaneQualityL_enum/1 -> Relational Operator4/1
  Constant4/1 -> Relational Operator4/2
  Relational Operator3/1 -> Logical Operator2/1
  Relational Operator4/1 -> Logical Operator2/2
  [dxR] -> Relational Operator5/1
  Constant6/1 -> Relational Operator5/2
  Relational Operator5/1 -> Logical Operator2/3
  Relational Operator6/1 -> Logical Operator2/4
  Switch/1 -> Unit Delay5/1, [C1RBias_new]  "C1RBias_new"
  Switch1/1 -> Unit Delay6/1, VPER_C1RBias_rad/1  "VPER_C1RBias_rad"
  [C1RBias_new] -> Abs2/1
  Abs2/1 -> Relational Operator6/1
  Constant7/1 -> Relational Operator6/2
  Forgetting_factor/1(C1R_Bias) -> Switch1/1  "C1L_Bias"
  [C1RBias_new] -> Forgetting_factor/1(C1RBias_new)
  Unit Delay5/1 -> Switch/3
  Unit Delay6/1 -> Switch1/3
  Abs3/1 -> Relational Operator3/1
  Logical Operator2/1 -> [Second_Condition_flg], Switch1/2
  Switch2/1 -> Add3/2
  Constant5/1 -> Switch2/1
  [reset_flag] -> Switch2/2
  Constant8/1 -> Switch3/1
  [reset_flag] -> Switch3/2
  Switch3/1 -> Add2/2
  Unit Delay7/1 -> [reset_flag]
  Unit Delay2/1 -> Switch3/3
  Unit Delay3/1 -> Switch2/3
  [First_Condition_flg] -> Logical Operator3/1
  [Second_Condition_flg] -> Logical Operator3/2
  Logical Operator3/1 -> Forgetting_factor/Enable
  [reset_flag] -> Switch4/2
  Constant2/1 -> Switch4/1
  Switch4/1 -> [dxR], Unit Delay3/1, Relational Operator2/1
  Add2/1 -> Switch5/3
  [reset_flag] -> Switch5/2
  Constant9/1 -> Switch5/1
  Switch5/1 -> divide/1, Unit Delay2/1
  Constant10/1 -> divide/3
  Constant11/1 -> divide1/3
  Constant3/1 -> divide2/1
  Gain/1 -> divide2/2
  Constant12/1 -> divide2/3

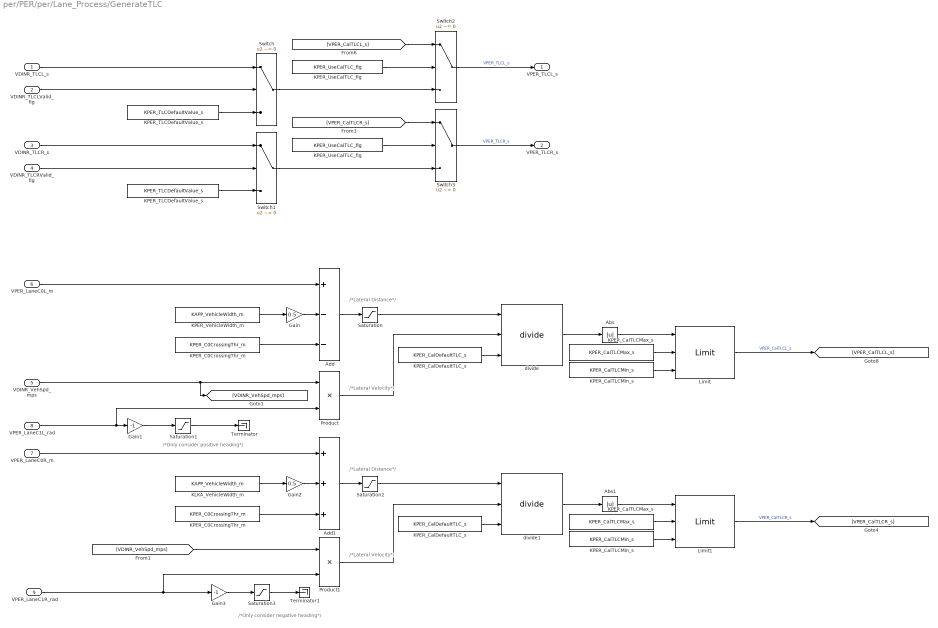
== system per/PER/per/Lane_Process/GenerateTLC ==
  note: /*Lateral Velocity*/
  note: /*Lateral Distance*/
  note: /*Only consider positive heading*/
  note: /*Only consider negative heading*/
  note: /*Lateral Distance*/
  note: /*Lateral Velocity*/
  VDINR_TLCL_s : Inport
  VDINR_TLCLValid_fig : Inport  Port=2
  VDINR_TLCR_s : Inport  Port=3
  VDINR_TLCRValid_fig : Inport  Port=4
  VDINR_VehSpd_mps : Inport  Port=5
  VPER_LaneC0L_m : Inport  Port=6
  VPER_LaneC0R_m : Inport  Port=7
  VPER_LaneC1L_rad : Inport  Port=8
  VPER_LaneC1R_rad : Inport  Port=9
  Abs : Abs
  Abs1 : Abs
  Add : Sum  Inputs=+--
  Add1 : Sum  Inputs=+++
  Gain : Gain  Gain=0.5
  Gain1 : Gain  Gain=-1
  Gain2 : Gain  Gain=0.5
  Gain3 : Gain  Gain=-1
  "KLKA_VehicleWidth_m " : Constant  Value=KAPP_VehicleWidth_m
  KPER_C0CrossingThr_m : Constant  Value=KPER_C0CrossingThr_m
  "KPER_C0CrossingThr_m " : Constant  Value=KPER_C0CrossingThr_m
  KPER_CalDefaultTLC_s : Constant  Value=KPER_CalDefaultTLC_s
  "KPER_CalDefaultTLC_s " : Constant  Value=KPER_CalDefaultTLC_s
  KPER_CalTLCMax_s : Constant  Value=KPER_CalTLCMax_s
  "KPER_CalTLCMax_s " : Constant  Value=KPER_CalTLCMax_s
  KPER_CalTLCMin_s : Constant  Value=KPER_CalTLCMin_s
  "KPER_CalTLCMin_s " : Constant  Value=KPER_CalTLCMin_s
  KPER_TLCDefaultValue_s : Constant  Value=KPER_TLCDefaultValue_s
  "KPER_TLCDefaultValue_s " : Constant  Value=KPER_TLCDefaultValue_s
  KPER_UseCalTLC_flg : Constant  Value=KPER_UseCalTLC_flg
  "KPER_UseCalTLC_flg " : Constant  Value=KPER_UseCalTLC_flg
  KPER_VehicleWidth_m : Constant  Value=KAPP_VehicleWidth_m
  Limit : hcu_lib/Limit  SystemSampleTime=-1
  Limit1 : hcu_lib/Limit  SystemSampleTime=-1
  Product : Product
  Product1 : Product
  Saturation : Saturate  UpperLimit=inf  LowerLimit=0
  Saturation1 : Saturate  UpperLimit=inf  LowerLimit=0
  Saturation2 : Saturate  UpperLimit=0  LowerLimit=-inf
  Saturation3 : Saturate  UpperLimit=0  LowerLimit=-inf
  Switch{,1..3} (4 alike) : Switch  Criteria=u2 ~= 0
  Terminator : Terminator
  Terminator1 : Terminator
  divide : hcu_lib/divide
  divide1 : hcu_lib/divide
  VPER_TLCL_s : Outport
  VPER_TLCR_s : Outport  Port=2
  wires:
  VDINR_TLCRValid_fig/1 -> Switch1/2
  Switch3/1 -> VPER_TLCR_s/1  "VPER_TLCR_s"
  "KPER_TLCDefaultValue_s "/1 -> Switch1/3
  Switch2/1 -> VPER_TLCL_s/1  "VPER_TLCL_s"
  KPER_TLCDefaultValue_s/1 -> Switch/3
  VDINR_TLCLValid_fig/1 -> Switch/2
  Gain/1 -> Add/2
  VPER_LaneC0L_m/1 -> Add/1
  KPER_VehicleWidth_m/1 -> Gain/1
  KPER_C0CrossingThr_m/1 -> Add/3
  VDINR_VehSpd_mps/1 -> Product/1, [VDINR_VehSpd_mps]
  Product/1 -> divide/2
  Add/1 -> Saturation/1
  KPER_CalDefaultTLC_s/1 -> divide/3
  Saturation/1 -> divide/1
  VPER_LaneC1L_rad/1 -> Product/2, Gain1/1
  Gain1/1 -> Saturation1/1
  divide/1 -> Abs/1
  KPER_CalTLCMax_s/1 -> Limit/2
  KPER_CalTLCMin_s/1 -> Limit/3
  Limit/1 -> [VPER_CalTLCL_s]  "VPER_CalTLCL_s"
  Saturation3/1 -> Terminator1/1
  Saturation2/1 -> divide1/1
  "KPER_CalDefaultTLC_s "/1 -> divide1/3
  Add1/1 -> Saturation2/1
  Product1/1 -> divide1/2
  [VDINR_VehSpd_mps] -> Product1/1
  "KPER_C0CrossingThr_m "/1 -> Add1/3
  "KLKA_VehicleWidth_m "/1 -> Gain2/1
  Gain2/1 -> Add1/2
  VPER_LaneC0R_m/1 -> Add1/1
  "KPER_CalTLCMax_s "/1 -> Limit1/2
  "KPER_CalTLCMin_s "/1 -> Limit1/3
  Limit1/1 -> [VPER_CalTLCR_s]  "VPER_CalTLCR_s"
  divide1/1 -> Abs1/1
  Gain3/1 -> Saturation3/1
  VPER_LaneC1R_rad/1 -> Product1/2, Gain3/1
  [VPER_CalTLCL_s] -> Switch2/1
  VDINR_TLCL_s/1 -> Switch/1
  VDINR_TLCR_s/1 -> Switch1/1
  [VPER_CalTLCR_s] -> Switch3/1
  KPER_UseCalTLC_flg/1 -> Switch2/2
  "KPER_UseCalTLC_flg "/1 -> Switch3/2
  Switch/1 -> Switch2/3
  Switch1/1 -> Switch3/3
  Saturation1/1 -> Terminator/1
  Abs/1 -> Limit/1
  Abs1/1 -> Limit1/1

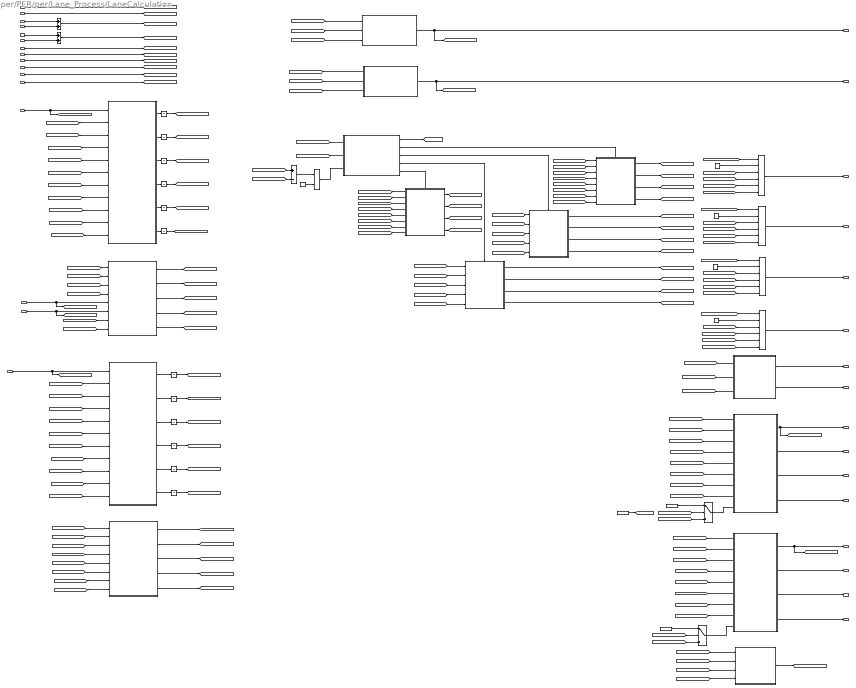
== system per/PER/per/Lane_Process/LaneCalculation ==
  VDINR_LaneC0L_m : Inport
  VDINR_LaneC0R_m : Inport  Port=2
  VDINR_LaneC1L_rad : Inport  Port=3
  VDINR_LaneC1R_rad : Inport  Port=4
  VDINR_LaneC2L_rat : Inport  Port=5
  VDINR_LaneC2R_rat : Inport  Port=6
  VDINR_LaneC3L_rat : Inport  Port=7
  VDINR_LaneC3R_rat : Inport  Port=8
  VDINR_YawRate_radps : Inport  Port=9
  VDINR_VehSpd_mps : Inport  Port=10
  VDINR_ViewRangeEndL_m : Inport  Port=11
  VDINR_ViewRangeEndR_m : Inport  Port=12
  VDINR_LaneQualityL_enum : Inport  Port=13
  VDINR_LaneQualityR_enum : Inport  Port=14
  VPER_C1LBias_rad : Inport  Port=15
  VPER_C1RBias_rad : Inport  Port=16
  Add : Sum
  Add1 : Sum
  Add2 : Sum  Inputs=+-
  C2diff_thr : Constant  Value=0.01
  Constant{,1..3} (4 alike) : Constant  Value=0  OutDataTypeStr=single
  GenerateLeftLane : Subsystem
  GenerateRightLane : Subsystem
  LR_Available : Subsystem  TreatAsAtomicUnit=on
  LR_NotAvailable : Subsystem  TreatAsAtomicUnit=on
  LaneL_estimator : Subsystem  TreatAsAtomicUnit=on
  LaneR_estimator : Subsystem  TreatAsAtomicUnit=on
  LaneResidual_Calculation : Subsystem
  LaneWidth : Subsystem
  Lane_Sw : Constant  Value=0
  Lane_status : Stateflow chart  TreatAsAtomicUnit=on
  LeftLaneAvail_flg : Constant
  Multiport Switch{,1..3} (4 alike) : MultiPortSwitch  DataPortOrder=Zero-based contiguous  Inputs=5
  OnlyL_Available : Subsystem  TreatAsAtomicUnit=on
  OnlyR_Available : Subsystem  TreatAsAtomicUnit=on
  Relational Operator : RelationalOperator  Operator=<=  OutDataTypeStr=boolean
  RightLaneAvail_flg : Constant
  Switch : Switch  Criteria=u2 ~= 0
  Switch1 : Switch  Criteria=u2 ~= 0
  Unit Delay{1,6..16} (12 alike) : UnitDelay  SampleTime=-1
  UsingRawLaneL : Subsystem
  UsingRawLaneR : Subsystem
  Using_estimator_LeftLane : Subsystem
  Using_estimator_RightLane : Subsystem
  "VPER_CenterLineC0_m " : Outport
  VPER_CenterLineC1_rad : Outport  Port=2
  VPER_CenterLineC2_rat : Outport  Port=3
  VPER_CenterLineC3_rat : Outport  Port=4
  VPER_LeftLaneAvail_flg : Outport  Port=5
  VPER_RightLaneAvail_flg : Outport  Port=6
  VPER_LaneC0L_m : Outport  Port=7
  VPER_LaneC1L_rad : Outport  Port=8
  VPER_LaneC2L_rat : Outport  Port=9
  VPER_LaneC3L_rat : Outport  Port=10
  VPER_LaneC0R_m : Outport  Port=11
  VPER_LaneC1R_rad : Outport  Port=12
  VPER_LaneC2R_rat : Outport  Port=13
  VPER_LaneC3R_rat : Outport  Port=14
  VPER_ResidualLaneL_s : Outport  Port=15
  VPER_ResidualLaneR_s : Outport  Port=16
  wires:
  [VDINR_LaneC0R_m] -> LR_Available/2(VDINR_LaneC0R_m)
  [VDINR_LaneC0L_m] -> LR_Available/1(VDINR_LaneC0L_m)
  [VDINR_LaneC2L_rat] -> OnlyL_Available/4(VDINR_LaneC2L_rat)
  OnlyL_Available/1(VPER_LCenterLineC0_m) -> [VPER_LCenterLineC0_m]
  [VDINR_LaneC3L_rat] -> OnlyL_Available/5(VDINR_LaneC3L_rat)
  LR_Available/1(VPER_RLCenterLineC0_m) -> [VPER_RLCenterLineC0_m]
  OnlyR_Available/1(VPER_RCenterLineC0_m) -> [VPER_RCenterLineC0_m]
  LR_Available/2(VPER_RLCenterLineC1_rad) -> [VPER_RLCenterLineC1_rad]
  OnlyR_Available/2(VPER_RCenterLineC1_rad) -> [VPER_RCenterLineC1_rad]
  [VPER_LaneWidth_m] -> OnlyL_Available/1(VPER_LaneWidth_m)
  OnlyR_Available/3(VPER_RCenterLineC2_rat) -> [VPER_RCenterLineC2_rat]
  OnlyR_Available/4(VPER_RCenterLineC3_rat) -> [VPER_RCenterLineC3_rat]
  [VPER_LaneWidth_m] -> OnlyR_Available/1(VPER_LaneWidth_m)
  LR_Available/3(VPER_RLCenterLineC2_rat) -> [VPER_RLCenterLineC2_rat]
  LR_Available/4(VPER_RLCenterLineC3_rat) -> [VPER_RLCenterLineC3_rat]
  [VDINR_LaneC0R_m] -> OnlyR_Available/2(VDINR_LaneC0R_m)
  [VDINR_LaneC0L_m] -> OnlyL_Available/2(VDINR_LaneC0L_m)
  [VDINR_LaneC1R_rad] -> OnlyR_Available/3(VDINR_LaneC1R_rad)
  [VDINR_LaneC2R_rat] -> OnlyR_Available/4(VDINR_LaneC2R_rat)
  [VDINR_LaneC3R_rat] -> OnlyR_Available/5(VDINR_LaneC3R_rat)
  OnlyL_Available/4(VPER_LCenterLineC3_rat) -> [VPER_LCenterLineC3_rat]
  OnlyL_Available/3(VPER_LCenterLineC2_rat) -> [VPER_LCenterLineC2_rat]
  OnlyL_Available/2(VPER_LCenterLineC1_rad) -> [VPER_LCenterLineC1_rad]
  [VDINR_LaneC1L_rad] -> OnlyL_Available/3(VDINR_LaneC1L_rad)
  [VDINR_LaneC3R_rat] -> LR_Available/8(VDINR_LaneC3R_rat)
  [VDINR_LaneC3L_rat] -> LR_Available/7(VDINR_LaneC3L_rat)
  [VDINR_LaneC2L_rat] -> LR_Available/5(VDINR_LaneC2L_rat)
  [VDINR_LaneC1R_rad] -> LR_Available/4(VDINR_LaneC1R_rad)
  [VDINR_LaneC1L_rad] -> LR_Available/3(VDINR_LaneC1L_rad)
  [VDINR_LaneC2R_rat] -> LR_Available/6(VDINR_LaneC2R_rat)
  VDINR_LaneC0L_m/1 -> [VDINR_LaneC0L_m]
  VDINR_LaneC0R_m/1 -> [VDINR_LaneC0R_m]
  VDINR_LaneC2L_rat/1 -> [VDINR_LaneC2L_rat]
  VDINR_LaneC2R_rat/1 -> [VDINR_LaneC2R_rat]
  VDINR_LaneC3L_rat/1 -> [VDINR_LaneC3L_rat]
  VDINR_LaneC3R_rat/1 -> [VDINR_LaneC3R_rat]
  VDINR_VehSpd_mps/1 -> [VDINR_VehSpd_mps], LaneL_estimator/6(VDINR_VehSpd_mps)
  Lane_status/1(SWCase) -> [SWCase]  "SW_CASE"
  Lane_status/2(LR_avail) -> LR_Available/Enable
  Lane_status/4(L_avail) -> OnlyL_Available/Enable
  Lane_status/3(R_avail) -> OnlyR_Available/Enable
  [SWCase] -> Multiport Switch/1
  [VPER_RLCenterLineC0_m] -> Multiport Switch/3
  [VPER_RCenterLineC0_m] -> Multiport Switch/4
  [VPER_LCenterLineC0_m] -> Multiport Switch/5
  Constant/1 -> Multiport Switch/2
  [SWCase] -> Multiport Switch1/1
  [VPER_RLCenterLineC1_rad] -> Multiport Switch1/3
  [VPER_RCenterLineC1_rad] -> Multiport Switch1/4
  [VPER_LCenterLineC1_rad] -> Multiport Switch1/5
  Constant1/1 -> Multiport Switch1/2
  [SWCase] -> Multiport Switch2/1
  Constant2/1 -> Multiport Switch2/2
  [VPER_RLCenterLineC2_rat] -> Multiport Switch2/3
  [VPER_RCenterLineC2_rat] -> Multiport Switch2/4
  [SWCase] -> Multiport Switch3/1
  Constant3/1 -> Multiport Switch3/2
  [VPER_RLCenterLineC3_rat] -> Multiport Switch3/3
  [VPER_RCenterLineC3_rat] -> Multiport Switch3/4
  [OptLaneC0L] -> LaneL_estimator/1(OptLaneC0L)
  [OptLaneC1L] -> LaneL_estimator/2(OptLaneC1L)
  [OptLaneC2L] -> LaneL_estimator/3(OptLaneC2L)
  [OptLaneC3L] -> LaneL_estimator/4(OptLaneC3L)
  VDINR_ViewRangeEndL_m/1 -> [VDINR_ViewRangeEndL_m]
  VDINR_ViewRangeEndR_m/1 -> [VDINR_ViewRangeEndR_m]
  [OptLaneC0R] -> LaneR_estimator/1(OptLaneC0R)
  [OptLaneC1R] -> LaneR_estimator/2(OptLaneC1R)
  [OptLaneC2R] -> LaneR_estimator/3(OptLaneC2R)
  [OptLaneC3R] -> LaneR_estimator/4(OptLaneC3R)
  [VDINR_YawRate_radps] -> LaneR_estimator/5(VDINR_YawRate_radps)
  [VDINR_VehSpd_mps] -> LaneR_estimator/6(VDINR_VehSpd_mps)
  Multiport Switch/1 -> "VPER_CenterLineC0_m "/1  "VPER_CenterLineC0_m"
  Multiport Switch1/1 -> VPER_CenterLineC1_rad/1  "VPER_CenterLineC1_rad"
  Multiport Switch2/1 -> VPER_CenterLineC2_rat/1  "VPER_CenterLineC2_rat"
  Multiport Switch3/1 -> VPER_CenterLineC3_rat/1  "VPER_CenterLineC3_rat"
  [VPER_LeftLaneAvail_flg] -> Lane_status/1(VPER_LeftLaneAvail_fig)
  [VPER_RightLaneAvail_flg] -> Lane_status/2(VPER_RightLaneAvail_fig)
  Lane_status/5(NO_avail) -> LR_NotAvailable/Enable
  [VPER_EstLaneC0L_m] -> LR_NotAvailable/1(VPER_EstLaneC0L_m)
  [VPER_EstLaneC0R_m] -> LR_NotAvailable/2(VPER_EstLaneC0R_m)
  [VPER_EstLaneC1L_rad] -> LR_NotAvailable/3(VPER_EstLaneC1L_rad)
  [VPER_EstLaneC1R_rad] -> LR_NotAvailable/4(VPER_EstLaneC1R_rad)
  [VPER_EstLaneC2R_rat] -> LR_NotAvailable/6(VPER_EstLaneC2R_rat)
  [VPER_EstLaneC3R_rat] -> LR_NotAvailable/8(VPER_EstLaneC3R_rat)
  [VPER_EstLaneC3L_rat] -> LR_NotAvailable/7(VPER_EstLaneC3L_rat)
  [VPER_EstLaneC2L_rat] -> LR_NotAvailable/5(VPER_EstLaneC2L_rat)
  LR_NotAvailable/1(VPER_EstCenterLineC0_m) -> [VPER_EstCenterLineC0_m]
  LR_NotAvailable/2(VPER_EstCenterLineC1_rad) -> [VPER_EstCenterLineC1_rad]
  LR_NotAvailable/3(VPER_EstCenterLineC2_rat) -> [VPER_EstCenterLineC2_rat]
  LR_NotAvailable/4(VPER_EstCenterLineC3_rat) -> [VPER_EstCenterLineC3_rat]
  [VPER_EstCenterLineC0_m] -> Multiport Switch/6
  LaneL_estimator/5(VPER_EstViewRangeEndL_m) -> [VPER_EstViewRangeEndL_m]
  LaneL_estimator/4(VPER_EstLaneC3L_rat) -> [VPER_EstLaneC3L_rat]
  LaneL_estimator/3(VPER_EstLaneC2L_rat) -> [VPER_EstLaneC2L_rat]
  LaneL_estimator/2(VPER_EstLaneC1L_rad) -> [VPER_EstLaneC1L_rad]
  LaneL_estimator/1(VPER_EstLaneC0L_m) -> [VPER_EstLaneC0L_m]
  [VPER_EstCenterLineC1_rad] -> Multiport Switch1/6
  [VPER_EstCenterLineC2_rat] -> Multiport Switch2/6
  [VPER_LCenterLineC2_rat] -> Multiport Switch2/5
  [VPER_EstCenterLineC3_rat] -> Multiport Switch3/6
  [VPER_LCenterLineC3_rat] -> Multiport Switch3/5
  [OptViewRange_L] -> LaneL_estimator/7(OptViewRange_L)
  [OptViewRange_R] -> LaneR_estimator/7(OptViewRange_R)
  [UsingRawLaneL_flg] -> LaneL_estimator/8(UsingRawLaneL_flg)
  [UsingRawLaneR_flg] -> LaneR_estimator/8(UsingRawLaneR_flg)
  VDINR_YawRate_radps/1 -> LaneL_estimator/5(VDINR_YawRate_radps), [VDINR_YawRate_radps]
  Using_estimator_LeftLane/1(VPER_LeftLaneAvail_flg) -> VPER_LeftLaneAvail_flg/1, [VPER_LeftLaneAvail_flg]
  [VDINR_LaneQualityL_enum] -> Using_estimator_LeftLane/1(VDINR_LaneQualityL_enum)
  [VDINR_ViewRangeEndL_m] -> Using_estimator_LeftLane/2(VDINR_ViewRangeEndL_m)
  [VPER_EstViewRangeEndL_m] -> Using_estimator_LeftLane/3(VPER_EstViewRangeEndL_m)
  VDINR_LaneQualityL_enum/1 -> [VDINR_LaneQualityL_enum], UsingRawLaneL/1(VDINR_LaneQualityL_enum)
  [VDINR_ViewRangeEndL_m] -> UsingRawLaneL/2(VDINR_ViewRangeEndL_m)
  [VPER_EstViewRangeEndL_m] -> UsingRawLaneL/3(VPER_EstViewRangeEndL_m)
  VDINR_LaneQualityR_enum/1 -> UsingRawLaneR/1(VDINR_LaneQualityR_enum), [VDINR_LaneQualityR_enum]
  Using_estimator_RightLane/1(VPER_RightLaneAvail_flg) -> [VPER_RightLaneAvail_flg], VPER_RightLaneAvail_flg/1
  [VDINR_LaneQualityR_enum] -> Using_estimator_RightLane/1(VDINR_LaneQualityR_enum)
  [VDINR_ViewRangeEndR_m] -> Using_estimator_RightLane/2(VDINR_ViewRangeEndR_m)
  [VPER_EstViewRangeEndR_m] -> Using_estimator_RightLane/3(VPER_EstViewRangeEndR_m)
  [VDINR_LaneC0L_m] -> GenerateLeftLane/1(VDINR_LaneC0L_m)
  [VPER_EstLaneC0L_m] -> GenerateLeftLane/2(VPER_EstLaneC0L_m)
  [VDINR_LaneC1L_rad] -> GenerateLeftLane/3(VDINR_LaneC1L_rad)
  [VPER_EstLaneC1L_rad] -> GenerateLeftLane/4(VPER_EstLaneC1L_rad)
  [VDINR_LaneC2L_rat] -> GenerateLeftLane/5(VDINR_LaneC2L_rat)
  [VPER_EstLaneC2L_rat] -> GenerateLeftLane/6(VPER_EstLaneC2L_rat)
  [VDINR_LaneC3L_rat] -> GenerateLeftLane/7(VDINR_LaneC3L_rat)
  [VPER_EstLaneC3L_rat] -> GenerateLeftLane/8(VPER_EstLaneC3L_rat)
  GenerateLeftLane/1(VPER_LaneC0L_m) -> [VPER_LaneC0L_m], VPER_LaneC0L_m/1
  GenerateLeftLane/2(VPER_LaneC1L_rad) -> VPER_LaneC1L_rad/1
  GenerateLeftLane/3(VPER_LaneC2L_rat) -> VPER_LaneC2L_rat/1
  GenerateLeftLane/4(VPER_LaneC3L_rat) -> VPER_LaneC3L_rat/1
  GenerateRightLane/1(VPER_LaneC0R_m) -> [VPER_LaneC0R_m], VPER_LaneC0R_m/1
  GenerateRightLane/2(VPER_LaneC1R_rad) -> VPER_LaneC1R_rad/1
  GenerateRightLane/3(VPER_LaneC2R_rat) -> VPER_LaneC2R_rat/1
  GenerateRightLane/4(VPER_LaneC3R_rat) -> VPER_LaneC3R_rat/1
  [VPER_EstLaneC1R_rad] -> GenerateRightLane/4(VPER_EstLaneC1R_rad)
  [VDINR_LaneC2R_rat] -> GenerateRightLane/5(VDINR_LaneC2R_rat)
  Switch1/1 -> GenerateRightLane/9(VPER_RightLaneAvail_flg)
  [VPER_EstLaneC3L_rat] -> GenerateRightLane/8(VPER_EstLaneC3R_rat)
  [VPER_EstLaneC2R_rat] -> GenerateRightLane/6(VPER_EstLaneC2R_rat)
  [VDINR_LaneC3R_rat] -> GenerateRightLane/7(VDINR_LaneC3R_rat)
  [VPER_EstLaneC0R_m] -> GenerateRightLane/2(VPER_EstLaneC0R_m)
  [VDINR_LaneC1R_rad] -> GenerateRightLane/3(VDINR_LaneC1R_rad)
  [VDINR_LaneC0R_m] -> GenerateRightLane/1(VDINR_LaneC0R_m)
  [VPER_EstLaneC0L_m] -> UsingRawLaneL/5(VPER_EstLaneC0L_m)
  [VDINR_LaneC0L_m] -> UsingRawLaneL/4(VDINR_LaneC0L_m)
  [VPER_EstLaneC1L_rad] -> UsingRawLaneL/7(VPER_EstLaneC1L_rad)
  [VDINR_LaneC1L_rad] -> UsingRawLaneL/6(VDINR_LaneC1L_rad)
  [VPER_EstLaneC2L_rat] -> UsingRawLaneL/9(VPER_EstLaneC2L_rat)
  [VDINR_LaneC2L_rat] -> UsingRawLaneL/8(VDINR_LaneC2L_rat)
  [VPER_EstLaneC3L_rat] -> UsingRawLaneL/11(VPER_EstLaneC3L_rat)
  [VDINR_LaneC3L_rat] -> UsingRawLaneL/10(VDINR_LaneC3L_rat)
  UsingRawLaneL/1(UsingRawLaneL_flg) -> Unit Delay11/1
  UsingRawLaneL/2(OptLaneC0L) -> Unit Delay6/1
  UsingRawLaneL/3(OptLaneC1L) -> Unit Delay7/1
  UsingRawLaneL/4(OptLaneC2L) -> Unit Delay8/1
  UsingRawLaneL/5(OptLaneC3L) -> Unit Delay9/1
  UsingRawLaneL/6(OptViewRange_L) -> Unit Delay10/1
  Unit Delay6/1 -> [OptLaneC0L]
  Unit Delay7/1 -> [OptLaneC1L]
  Unit Delay8/1 -> [OptLaneC2L]
  Unit Delay9/1 -> [OptLaneC3L]
  Unit Delay10/1 -> [OptViewRange_L]
  Unit Delay11/1 -> [UsingRawLaneL_flg]
  [VDINR_ViewRangeEndR_m] -> UsingRawLaneR/2(VDINR_ViewRangeEndR_m)
  [VPER_EstViewRangeEndR_m] -> UsingRawLaneR/3(VPER_EstViewRangeEndR_m)
  UsingRawLaneR/1(UsingRawLaneR_flg) -> Unit Delay12/1
  Unit Delay12/1 -> [UsingRawLaneR_flg]
  [VPER_EstLaneC0R_m] -> UsingRawLaneR/5(VPER_EstLaneC0R_m)
  [VDINR_LaneC0R_m] -> UsingRawLaneR/4(VDINR_LaneC0R_m)
  [VPER_EstLaneC1R_rad] -> UsingRawLaneR/7(VPER_EstLaneC1R_rad)
  [VDINR_LaneC1R_rad] -> UsingRawLaneR/6(VDINR_LaneC1R_rad)
  [VDINR_LaneC2R_rat] -> UsingRawLaneR/8(VDINR_LaneC2R_rat)
  [VPER_EstLaneC2R_rat] -> UsingRawLaneR/9(VPER_EstLaneC2R_rat)
  [VDINR_LaneC3R_rat] -> UsingRawLaneR/10(VDINR_LaneC3R_rat)
  [VPER_EstLaneC3R_rat] -> UsingRawLaneR/11(VPER_EstLaneC3R_rat)
  UsingRawLaneR/2(OptLaneC0R) -> Unit Delay13/1
  UsingRawLaneR/3(OptLaneC1R) -> Unit Delay14/1
  UsingRawLaneR/4(OptLaneC2R) -> Unit Delay15/1
  UsingRawLaneR/5(OptLaneC3R) -> Unit Delay16/1
  Unit Delay13/1 -> [OptLaneC0R]
  Unit Delay14/1 -> [OptLaneC1R]
  Unit Delay15/1 -> [OptLaneC2R]
  Unit Delay16/1 -> [OptLaneC3R]
  LaneR_estimator/1(VPER_EstLaneC0R_m) -> [VPER_EstLaneC0R_m]
  LaneR_estimator/2(VPER_EstLaneC1R_rad) -> [VPER_EstLaneC1R_rad]
  LaneR_estimator/3(VPER_EstLaneC2R_rat) -> [VPER_EstLaneC2R_rat]
  LaneR_estimator/4(VPER_EstLaneC3R_rat) -> [VPER_EstLaneC3R_rat]
  LaneR_estimator/5(VPER_EstViewRangeEndR_m) -> [VPER_EstViewRangeEndR_m]
  UsingRawLaneR/6(OptViewRange_R) -> Unit Delay1/1
  Unit Delay1/1 -> [OptViewRange_R]
  [VPER_LeftLaneAvail_flg] -> LaneWidth/1(VPER_LeftLaneAvail_flg)
  [VPER_RightLaneAvail_flg] -> LaneWidth/2(VPER_RightLaneAvail_flg)
  [VPER_LaneC0R_m] -> LaneWidth/4(VDINR_LaneC0R_m)
  [VPER_LaneC0L_m] -> LaneWidth/3(VDINR_LaneC0L_m)
  LaneWidth/1(VPER_LaneWidth_m) -> [VPER_LaneWidth_m]
  VDINR_LaneC1L_rad/1 -> Add/1
  VPER_C1LBias_rad/1 -> Add/2
  Add/1 -> [VDINR_LaneC1L_rad]
  VDINR_LaneC1R_rad/1 -> Add1/1
  VPER_C1RBias_rad/1 -> Add1/2
  Add1/1 -> [VDINR_LaneC1R_rad]
  [VPER_EstViewRangeEndL_m] -> LaneResidual_Calculation/1(VPER_EstViewRangeEndL_m)
  [VDINR_VehSpd_mps] -> LaneResidual_Calculation/2(VDINR_VehSpd_mps)
  [VPER_EstViewRangeEndR_m] -> LaneResidual_Calculation/3(VPER_EstViewRangeEndR_m)
  LaneResidual_Calculation/1(VPER_ResidualLaneL_s) -> VPER_ResidualLaneL_s/1
  LaneResidual_Calculation/2(VPER_ResidualLaneR_s) -> VPER_ResidualLaneR_s/1
  [VDINR_LaneC2L_rat] -> Add2/1
  [VDINR_LaneC2R_rat] -> Add2/2
  Add2/1 -> Relational Operator/1
  C2diff_thr/1 -> Relational Operator/2
  Relational Operator/1 -> Lane_status/3(VPER_C2Diff_flg)
  Switch/1 -> GenerateLeftLane/9(VPER_LeftLaneAvail_flg)
  [Lane_Sw] -> Switch/2
  [VPER_LeftLaneAvail_flg] -> Switch/3
  LeftLaneAvail_flg/1 -> Switch/1
  Lane_Sw/1 -> [Lane_Sw]
  [Lane_Sw] -> Switch1/2
  [VPER_RightLaneAvail_flg] -> Switch1/3
  RightLaneAvail_flg/1 -> Switch1/1

== system per/PER/per/Lane_Process/C1L_Bias/Forgetting_factor ==
  C1LBias_new : Inport
  Enable : EnablePort
  FF : Stateflow chart  TreatAsAtomicUnit=on
  Forget_factor : Constant  Value=0.99933  OutDataTypeStr=single
  Terminator : Terminator
  C1L_Bias : Outport
  wires:
  C1LBias_new/1 -> FF/1(C1LBias_new)
  FF/1(C1L_Bias) -> C1L_Bias/1
  FF/2(P_L) -> Terminator/1
  Forget_factor/1 -> FF/2(Forget_Factor)

== system per/PER/per/Lane_Process/C1R_Bias/Forgetting_factor ==
  C1RBias_new : Inport
  Enable : EnablePort
  FF : Stateflow chart  TreatAsAtomicUnit=on
  Forget_factor : Constant  Value=0.99933  OutDataTypeStr=single
  Terminator : Terminator
  C1R_Bias : Outport
  wires:
  C1RBias_new/1 -> FF/1(C1RBias_new)
  FF/1(C1R_Bias) -> C1R_Bias/1
  FF/2(P_R) -> Terminator/1
  Forget_factor/1 -> FF/2(Forget_Factor)

== system per/PER/per/Lane_Process/LaneCalculation/GenerateLeftLane ==
  VDINR_LaneC0L_m : Inport
  VPER_EstLaneC0L_m : Inport  Port=2
  VDINR_LaneC1L_rad : Inport  Port=3
  VPER_EstLaneC1L_rad : Inport  Port=4
  VDINR_LaneC2L_rat : Inport  Port=5
  VPER_EstLaneC2L_rat : Inport  Port=6
  VDINR_LaneC3L_rat : Inport  Port=7
  VPER_EstLaneC3L_rat : Inport  Port=8
  VPER_LeftLaneAvail_flg : Inport  Port=9
  Switch{3,12..14} (4 alike) : Switch  Criteria=u2 ~= 0
  VPER_LaneC0L_m : Outport
  VPER_LaneC1L_rad : Outport  Port=2
  VPER_LaneC2L_rat : Outport  Port=3
  VPER_LaneC3L_rat : Outport  Port=4
  wires:
  VPER_EstLaneC0L_m/1 -> Switch3/3
  Switch12/1 -> VPER_LaneC1L_rad/1  "VPER_LaneC1L_rad"
  VPER_EstLaneC1L_rad/1 -> Switch12/3
  VDINR_LaneC1L_rad/1 -> Switch12/1
  Switch3/1 -> VPER_LaneC0L_m/1  "VPER_LaneC0L_m"
  Switch13/1 -> VPER_LaneC2L_rat/1  "VPER_LaneC2L_rat"
  VPER_EstLaneC2L_rat/1 -> Switch13/3
  VDINR_LaneC2L_rat/1 -> Switch13/1
  VPER_LeftLaneAvail_flg/1 -> Switch14/2, Switch13/2, Switch12/2, Switch3/2
  VPER_EstLaneC3L_rat/1 -> Switch14/3
  VDINR_LaneC3L_rat/1 -> Switch14/1
  VDINR_LaneC0L_m/1 -> Switch3/1
  Switch14/1 -> VPER_LaneC3L_rat/1  "VPER_LaneC3L_rat"
